simulink model "shuntdcmotorstartwithresistanceproject"  (R2023b)
settings: Solver=VariableStepAuto  StartTime=0.0  StopTime=10.0  RelTol=1e-3
undefined symbols (not defined in the file): D, J, Laq, Ra
libraries: simulink_extras x3, simulink x1, hdlsllib x1
settings Model: Creator=HP  LastModifiedBy=HP

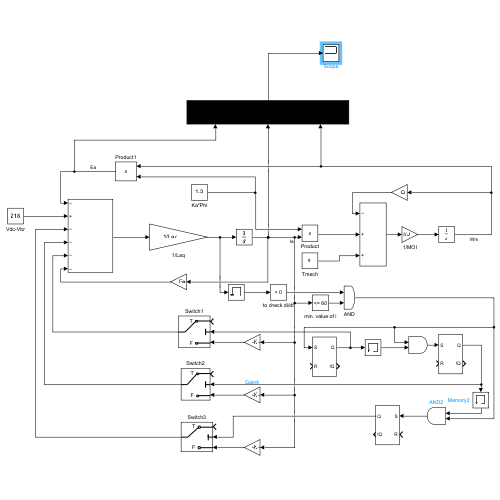
[thumbnail: Simulink's stored preview of the top-level diagram]
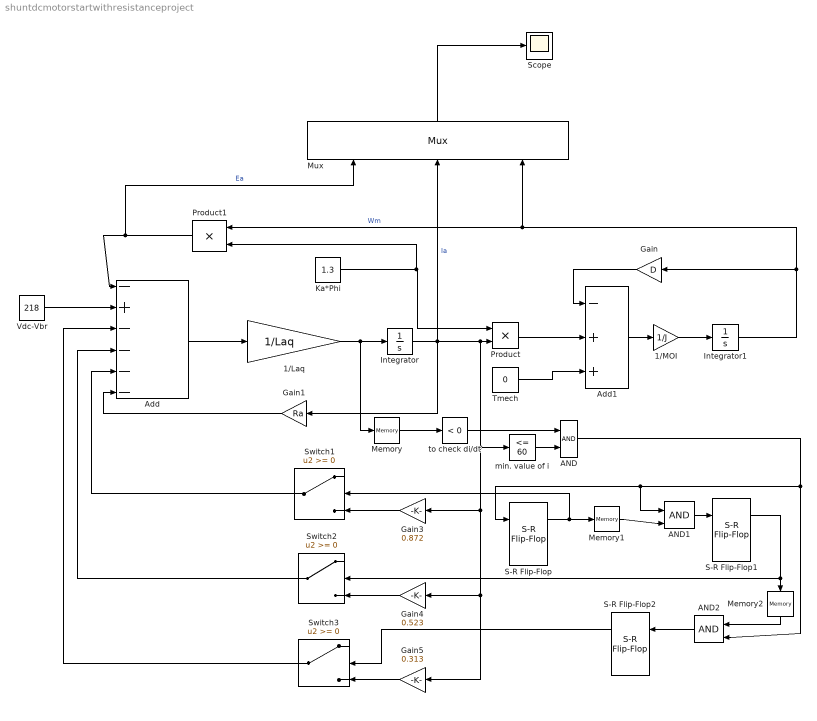
== system shuntdcmotorstartwithresistanceproject ==
  1/Laq : Gain  Gain=1/Laq
  1/MOI : Gain  Gain=1/J
  AND : Logic  IconShape=distinctive  AllPortsSameDT=off  OutDataTypeStr=boolean
  AND1 : Logic  IconShape=distinctive  AllPortsSameDT=off  OutDataTypeStr=boolean
  AND2 : Logic  IconShape=distinctive  AllPortsSameDT=off  OutDataTypeStr=boolean
  Add : Sum  Inputs=-+----
  Add1 : Sum  Inputs=-++
  Gain : Gain  Gain=D
  Gain1 : Gain  Gain=Ra
  Gain3 : Gain  Gain=0.872
  Gain4 : Gain  Gain=0.523
  Gain5 : Gain  Gain=0.313
  Integrator : Integrator
  Integrator1 : Integrator
  Ka*Phi : Constant  Value=1.3
  Memory : Memory
  Memory1 : Memory
  Memory2 : Memory
  Mux : Mux  Inputs=3
  Product : Product
  Product1 : Product
  S-R Flip-Flop : simulink_extras/Flip Flops/S-R Flip-Flop  initial_condition=0
  S-R Flip-Flop1 : simulink_extras/Flip Flops/S-R Flip-Flop  initial_condition=0
  S-R Flip-Flop2 : simulink_extras/Flip Flops/S-R Flip-Flop  initial_condition=0
  Scope : Scope
  Switch1 : Switch  SaturateOnIntegerOverflow=off  InputSameDT=off
  Switch2 : Switch  SaturateOnIntegerOverflow=off  InputSameDT=off
  Switch3 : Switch  SaturateOnIntegerOverflow=off  InputSameDT=off
  Tmech : Constant  Value=0
  Vdc-Vbr : Constant  Value=218
  min. value of i : simulink/Logic and Bit Operations/Compare To Constant  relop=<=  const=60  OutDataTypeStr=boolean
  to check di/dt : hdlsllib/Logic and Bit Operations/Compare To Zero  relop=<  OutDataTypeStr=boolean
  wires:
  Vdc-Vbr/1 -> Add/2
  Add/1 -> 1/Laq/1
  1/Laq/1 -> Memory/1, Integrator/1
  Integrator/1 -> Gain5/1, Gain4/1, Gain3/1, min. value of i/1, Product/2, Mux/2, Gain1/1  "Ia"
  Ka*Phi/1 -> Product1/2, Product/1
  Product/1 -> Add1/2
  Tmech/1 -> Add1/3
  Add1/1 -> 1/MOI/1
  1/MOI/1 -> Integrator1/1
  Integrator1/1 -> Mux/3, Product1/1, Gain/1  "Wm"
  Gain/1 -> Add1/1
  Product1/1 -> Mux/1, Add/1  "Ea"
  Mux/1 -> Scope/1
  Memory/1 -> to check di/dt/1
  to check di/dt/1 -> AND/1
  min. value of i/1 -> AND/2
  AND/1 -> AND2/2, AND1/1, S-R Flip-Flop/1
  S-R Flip-Flop/1 -> Switch1/2, Memory1/1
  Memory1/1 -> AND1/2
  AND1/1 -> S-R Flip-Flop1/1
  S-R Flip-Flop1/1 -> Memory2/1, Switch2/2
  Memory2/1 -> AND2/1
  AND2/1 -> S-R Flip-Flop2/1
  Gain3/1 -> Switch1/3
  Gain4/1 -> Switch2/3
  Gain5/1 -> Switch3/3
  S-R Flip-Flop2/1 -> Switch3/2
  Switch1/1 -> Add/5
  Switch2/1 -> Add/4
  Switch3/1 -> Add/3
  Gain1/1 -> Add/6
